simulink model "fz_estimator"  (R2024b)
settings: Solver=FixedStepAuto  StartTime=0.0  StopTime=10.0  RelTol=1e-3
model workspace (MAT data in the model file):
  dt = Simulink.Parameter
  dt.Value = 0.004
  dt.Complexity = 'real'
  dt.Dimensions = [1 1]
  dt.DataType = 'double'
values from neighbouring files (symbols this model uses):
  dt = 0.01    [ekf_test.m]
undefined symbols (not defined in the file or in its folder): Discrete, Time
libraries: ctrlSharedLib x1
settings Model: Creator=lukec  LastModifiedBy=lukec
settings OptimizationCC: DefaultParameterBehavior=Inlined  EnhancedBackFolding=on  PassReuseOutputArgsAs=Individual arguments  ZeroExternalMemoryAtStartup=off  ZeroInternalMemoryAtStartup=off  OptimizeBlockOrder=speed  DifferentSizesBufferReuse=on  OptimizationCustomize=off  EfficientTunableParamExpr=on
settings DebuggingCC: ParameterTunabilityLossMsg=error
settings HardwareCC: ProdBitPerPointer=32  ProdBitPerSizeT=32  ProdBitPerPtrDiffT=32  ProdLargestAtomicInteger=Long  ProdLargestAtomicFloat=Double  ProdWordSize=32  ProdHWDeviceType=ARM Compatible->ARM Cortex-M
settings SFSimCC: MATLABDynamicMemAlloc=off
settings RTWCC: Description=Embedded Coder  SystemTargetFile=ert.tlc  GenCodeOnly=on  PackageGeneratedCodeAndArtifacts=on  TemplateMakefile=ert_default_tmf  Toolchain=CMake  TargetLang=C++  HalideCodeGeneration=on
settings CodeAppCC: ForceParamTrailComments=on  IgnoreCustomStorageClasses=off  MaxIdLength=255  OperatorAnnotations=on  SimulinkDataObjDesc=on  SFDataObjDesc=on  InsertBlockDesc=on
settings ERTTargetCC: TargetLangStandard=C++17 (ISO)  CodeInterfacePackaging=C++ class  RootIOFormat=Structure reference  ERTCustomFileTemplate=example_file_process.tlc  ArrayContainerType=std::array

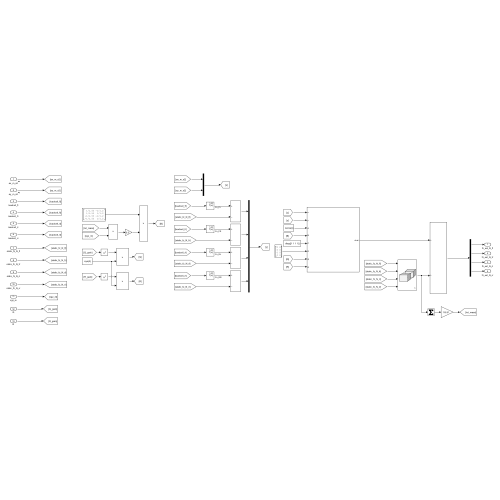
[thumbnail: Simulink's stored preview of the top-level diagram]
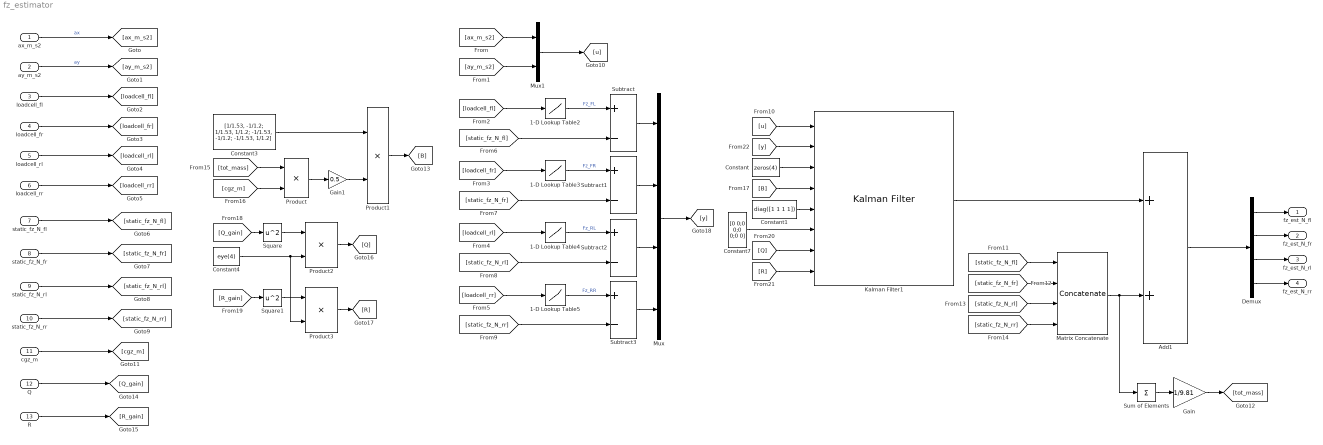
== system fz_estimator ==
  ax_m_s2 : Inport
  ay_m_s2 : Inport  Port=2
  loadcell_fl : Inport  Port=3
  loadcell_fr : Inport  Port=4
  loadcell_rl : Inport  Port=5
  loadcell_rr : Inport  Port=6
  static_fz_N_fl : Inport  Port=7
  static_fz_N_fr : Inport  Port=8
  static_fz_N_rl : Inport  Port=9
  static_fz_N_rr : Inport  Port=10
  cgz_m : Inport  Port=11
  Q : Inport  Port=12
  R : Inport  Port=13
  1-D Lookup Table2 : Lookup_n-D  NumberOfTableDimensions=1  BreakpointsForDimension1=[0 71 227 264 464 569 704 797 909 1076 1234]  Table=[0 11.8 22.2 37.5 63.2 79 102.1 120.3 133 154 174].*4.448  InternalRulePriority=Speed  RndMeth=Simplest
  1-D Lookup Table3 : Lookup_n-D  NumberOfTableDimensions=1  BreakpointsForDimension1=[0 6 207 312 449 547 666 709 803 969]  Table=[0 31.1 57.9 74.4 100.3 117 129.5 134 143 167.8].*4.448  InternalRulePriority=Speed  RndMeth=Simplest
  1-D Lookup Table4 : Lookup_n-D  NumberOfTableDimensions=1  BreakpointsForDimension1=[0 122 148 266 351 429 511 565 661 767 900 1023]  Table=[0 28.1 33 50.6 64.7 81 96.4 107.3 123.2 139.5 160.5 180.5].*4.448  InternalRulePriority=Speed  RndMeth=Simplest
  1-D Lookup Table5 : Lookup_n-D  NumberOfTableDimensions=1  BreakpointsForDimension1=[0 682 830 847]  Table=[0 108.9 137.9 142.5].*4.448  InternalRulePriority=Speed  RndMeth=Simplest
  Add1 : Sum
  Constant : Constant  Value=zeros(4)
  Constant1 : Constant  Value=diag([1 1 1 1])
  Constant3 : Constant  Value=[1/1.53, -1/1.2; 1/1.53, 1/1.2; -1/1.53, -1/1.2; -1/1.53, 1/1.2]
  Constant4 : Constant  Value=eye(4)
  Constant7 : Constant  Value=[0 0;0 0;0 0;0 0]
  Demux : Demux
  Gain : Gain  Gain=1/9.81
  Gain1 : Gain  Gain=0.5
  Kalman Filter1 : ctrlSharedLib/Kalman Filter  TimeDomain=Discrete-Time  UseCurrentEstimator=on  ModelSource=Input port  ModelSourceVariable=ss(0.95,1,1,0,1)  A=zeros(4)  B=(260*0.277/2)*[1/1.53, -1/1.2; 1/1.53, 1/1.2; -1/1.53, -1/1.2; -1/1.53, 1/1.2]  C=diag([1 1 1 1])  D=0  NumberOfStates=4  NumberOfInputs=2  NumberOfOutputs=4  InitialEstimateSource=Dialog  X0=zeros(4, 1)  P0=10  UseK=off  UseGH=off  NumberOfProcessNoiseInputs=1  G=1  TimeInvariantG=on  H=0  TimeInvariantH=on  Q=(120^2)*eye(4);  TimeInvariantQ=off  R=(70^2)*eye(4);  TimeInvariantR=off  N=0  TimeInvariantN=on  AddInputPort=on  AddEnablePort=off  OutputEstimatedY=off  OutputP=off  Ts=dt
  Matrix Concatenate : Concatenate  NumInputs=4  Mode=Multidimensional array
  Mux : Mux
  Mux1 : Mux  Inputs=2
  Product{,1..3} (4 alike) : Product
  Square : Math  Operator=square
  Square1 : Math  Operator=square
  Subtract{,1..3} (4 alike) : Sum  Inputs=+-
  Sum of Elements : Sum  Inputs=+
  fz_est_N_fl : Outport
  fz_est_N_fr : Outport  Port=2
  fz_est_N_rl : Outport  Port=3
  fz_est_N_rr : Outport  Port=4
  wires:
  1-D Lookup Table4/1 -> Subtract2/1  "Fz_RL"
  Matrix Concatenate/1 -> Sum of Elements/1, Add1/2
  Subtract2/1 -> Mux/3
  Subtract3/1 -> Mux/4
  Mux/1 -> [y]
  Kalman Filter1/1 -> Add1/1
  1-D Lookup Table5/1 -> Subtract3/1  "Fz_RR"
  Subtract1/1 -> Mux/2
  [loadcell_fl] -> 1-D Lookup Table2/1
  1-D Lookup Table2/1 -> Subtract/1  "Fz_FL"
  Subtract/1 -> Mux/1
  Add1/1 -> Demux/1
  [loadcell_rr] -> 1-D Lookup Table5/1
  [loadcell_fr] -> 1-D Lookup Table3/1
  [loadcell_rl] -> 1-D Lookup Table4/1
  1-D Lookup Table3/1 -> Subtract1/1  "Fz_FR"
  ax_m_s2/1 -> [ax_m_s2]  "ax"
  ay_m_s2/1 -> [ay_m_s2]  "ay"
  loadcell_fl/1 -> [loadcell_fl]
  loadcell_rr/1 -> [loadcell_rr]
  loadcell_rl/1 -> [loadcell_rl]
  loadcell_fr/1 -> [loadcell_fr]
  static_fz_N_fr/1 -> [static_fz_N_fr]
  static_fz_N_fl/1 -> [static_fz_N_fl]
  static_fz_N_rr/1 -> [static_fz_N_rr]
  static_fz_N_rl/1 -> [static_fz_N_rl]
  [ax_m_s2] -> Mux1/1
  [ay_m_s2] -> Mux1/2
  Mux1/1 -> [u]
  [static_fz_N_fl] -> Subtract/2
  [static_fz_N_fr] -> Subtract1/2
  [static_fz_N_rl] -> Subtract2/2
  [static_fz_N_rr] -> Subtract3/2
  [u] -> Kalman Filter1/1
  [static_fz_N_fl] -> Matrix Concatenate/1
  [static_fz_N_fr] -> Matrix Concatenate/2
  [static_fz_N_rl] -> Matrix Concatenate/3
  [static_fz_N_rr] -> Matrix Concatenate/4
  Demux/1 -> fz_est_N_fl/1
  Demux/2 -> fz_est_N_fr/1
  Demux/3 -> fz_est_N_rl/1
  Demux/4 -> fz_est_N_rr/1
  Constant/1 -> Kalman Filter1/3
  Constant1/1 -> Kalman Filter1/5
  Constant7/1 -> Kalman Filter1/6
  cgz_m/1 -> [cgz_m]
  Sum of Elements/1 -> Gain/1
  Gain/1 -> [tot_mass]
  [B] -> Kalman Filter1/4
  Q/1 -> [Q_gain]
  R/1 -> [R_gain]
  [Q_gain] -> Square/1
  Square/1 -> Product2/1
  Product2/1 -> [Q]
  Product3/1 -> [R]
  Square1/1 -> Product3/1
  Constant4/1 -> Product2/2, Product3/2
  [R_gain] -> Square1/1
  [cgz_m] -> Product/2
  Product1/1 -> [B]
  [tot_mass] -> Product/1
  Constant3/1 -> Product1/1
  Product/1 -> Gain1/1
  Gain1/1 -> Product1/2
  [Q] -> Kalman Filter1/7
  [R] -> Kalman Filter1/8
  [y] -> Kalman Filter1/2
